simulink model "model2"  (R2021b)
settings: Solver=VariableStepAuto  StartTime=0.0  StopTime=300  RelTol=1e-3
undefined symbols (not defined in the file): k, r, T, tau
settings Model: Creator=szczy  LastModifiedBy=szczy

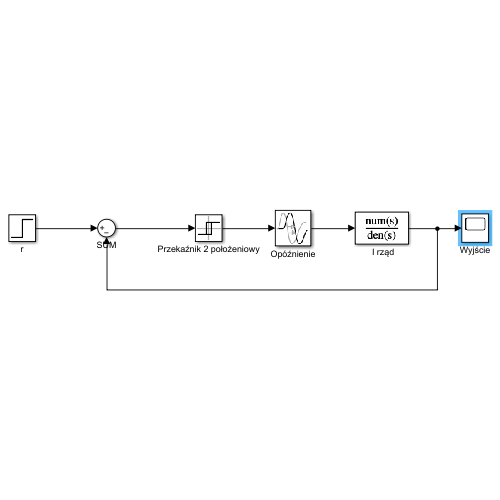
[thumbnail: Simulink's stored preview of the top-level diagram]
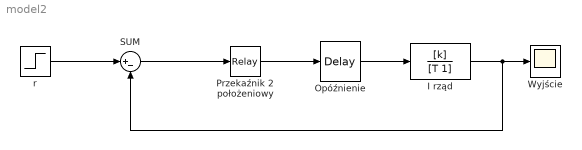
== system model2 ==
  " I rząd" : TransferFcn  Numerator=[k]  Denominator=[T 1]
  Opóźnienie : TransportDelay  DelayTime=tau
  Przekaźnik 2 położeniowy : Relay  OnOutputValue=5  OffOutputValue=1
  SUM : Sum  Inputs=|+-
  Wyjście : Scope
  r : Step  After=r  SampleTime=0
  wires:
  r/1 -> SUM/1
  " I rząd"/1 -> SUM/2, Wyjście/1
  Opóźnienie/1 -> " I rząd"/1
  SUM/1 -> Przekaźnik 2 położeniowy/1
  Przekaźnik 2 położeniowy/1 -> Opóźnienie/1
